simulink model "BD_PAR"  (Simulink 10.1)
settings: Solver=ode1  StartTime=0.0  StopTime=max(cyc_mph(:,1))  FixedStep=1  MaxStep=1  RelTol=1e-3  AbsTol=1e-3
undefined symbols (not defined in the file): ess_on, ex_calc, fc_emis, fc_max_trq, fc_trq_scale, vc_idle_bool, vc_idle_spd
libraries: lib_transmission x4, lib_wheel x2, lib_help x2, lib_accessory x2, lib_controls x2, lib_outputs x1, lib_interactive x1, lib_drive_cycle x1, lib_energy_storage x1, lib_exhaust x1, lib_fuel_converter x1, lib_electric_machine x1
settings Model: Creator=mokeefe  LastModifiedBy=sateeshk  ExtModeTrigMode=oneshot  ExtModeArmWhenConnect=off
settings SolverCC: AutoScaleAbsTol=off
settings DataIOCC: SignalLoggingSaveFormat=ModelDataLogs  SaveOutput=off  SaveTime=off
settings OptimizationCC: BooleanDataType=off  ExpressionDepthLimit=2147483647
settings DebuggingCC: SaveWithParameterizedLinksMsg=none  SignalResolutionControl=TryResolveAllWithWarning  MultiTaskDSMMsg=warning  MultiTaskCondExecSysMsg=none  FcnCallInpInsideContextMsg=warning  UnconnectedLineMsg=none  StateNameClashWarn=warning
settings HardwareCC: TargetUnknown=on
settings RTWCC: TemplateMakefile=grt_vc.tmf

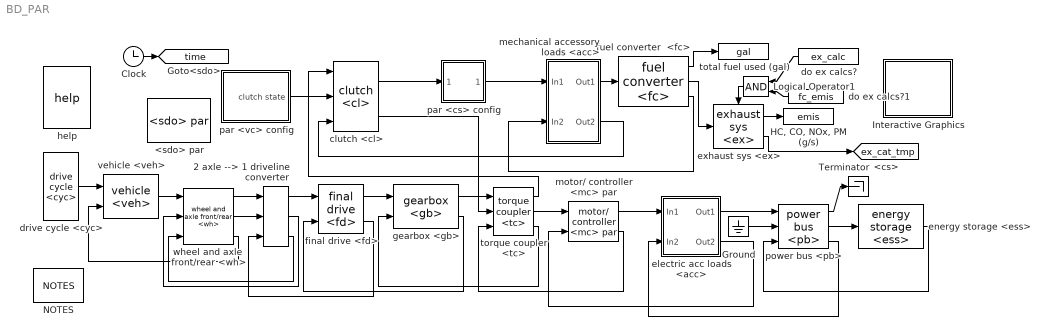
== system BD_PAR ==
  2 axle --> 1 driveline converter : lib_wheel/2 axle --> 1 driveline converter  SystemSampleTime=-1  Latency=0  AutoFrameSizeCalculation=off
  <sdo> par : lib_outputs/<sdo> par  SystemSampleTime=-1  Latency=0  AutoFrameSizeCalculation=off
  Clock : Clock
  Ground : Ground
  "HC, CO, NOx, PM (g/s)" : ToWorkspace  VariableName=emis
  Interactive Graphics : Subsystem  BlockChoice=off
      settings: AttributesFormatString=%<BlockChoice>  TemplateBlock=lib_interactive/Interactive Graphics  MemberBlocks=off,on
  Logical Operator1 : Logic
  NOTES : lib_help/NOTES  SystemSampleTime=-1  Latency=0  AutoFrameSizeCalculation=off
  Terminator : Terminator
  clutch <cl> : lib_transmission/clutch <cl>  slip_spd=vc_launch_spd  maxtrq=max(fc_max_trq)*fc_trq_scale
  do ex calcs? : Constant  Value=ex_calc
  do ex calcs?1 : Constant  Value=fc_emis
  drive cycle <cyc> : lib_drive_cycle/drive cycle <cyc>  SystemSampleTime=-1  Latency=0  AutoFrameSizeCalculation=off
  electric acc loads <acc> : Subsystem
      mask Display: image(imread('bdi_acc_elec.bmp'))
  energy storage <ess> : lib_energy_storage/energy storage <ess>  SystemSampleTime=-1  Latency=0  AutoFrameSizeCalculation=off
      link override ess config: BlockChoice=energy storage <ess>
  exhaust sys <ex> : lib_exhaust/exhaust sys <ex>  SystemSampleTime=-1  Latency=0  AutoFrameSizeCalculation=off
  final drive <fd> : lib_transmission/final drive <fd>  SystemSampleTime=-1  Latency=0  AutoFrameSizeCalculation=off
  fuel converter  <fc> : lib_fuel_converter/fuel converter  <fc>  SystemSampleTime=-1  Latency=0  AutoFrameSizeCalculation=off
      link override fuel use and EO emis Configurable Subsystem: BlockChoice=fuel use and EO emis
  gearbox <gb> : lib_transmission/gearbox <gb>  SystemSampleTime=-1  Latency=0  AutoFrameSizeCalculation=off
  help : lib_help/help  SystemSampleTime=-1  Latency=0  AutoFrameSizeCalculation=off
  mechanical accessory loads <acc> : Subsystem
      mask Display: image(imread('bdi_acc_pic.bmp'))
  motor/ controller <mc> par : lib_electric_machine/motor// controller <mc> par  SystemSampleTime=-1  Latency=0  AutoFrameSizeCalculation=off
  par <cs> config : Subsystem  BlockChoice=electric assist control strategy <cs>
      settings: AttributesFormatString=%<BlockChoice>  TemplateBlock=lib_controls/par <cs> config  MemberBlocks=Adaptive control strategy <cs>,Fuzzy Logic control strategy <cs>,Fuzzy Logic control strategy with Emissions <cs>,electric assist control strategy <cs>,electric assist control strategy bal <cs>
  par <vc> config : Subsystem  BlockChoice=<vc> par
      link override <vc> par Adaptive/config traction control: BlockChoice=traction control
      link override <vc> par/config traction control: BlockChoice=traction control 2 axle
      settings: AttributesFormatString=%<BlockChoice>  TemplateBlock=lib_controls/par <vc> config  MemberBlocks=<vc> par,<vc> par Adaptive,<vc> par balanced
  power bus <pb> : lib_power_bus/power bus <pb>  SystemSampleTime=-1  Latency=0  AutoFrameSizeCalculation=off
  torque coupler <tc> : lib_transmission/torque coupler <tc>  SystemSampleTime=-1  Latency=0  AutoFrameSizeCalculation=off
  total fuel used (gal) : ToWorkspace  VariableName=gal
  vehicle <veh> : lib_vehicle/vehicle <veh>  SystemSampleTime=-1  Latency=0  AutoFrameSizeCalculation=off
      link override record achieved force outputs/rolling resistance force: BlockChoice=force req'd to overcome rolling resistance (N)
      link override rolling resistance force: BlockChoice=force req'd to overcome rolling resistance (N)
      link override vehicle speed: BlockChoice=vehicle speed (m/s)
  wheel and axle  front/rear <wh> : lib_wheel/wheel and axle  front//rear <wh>  SystemSampleTime=-1  Latency=0  AutoFrameSizeCalculation=off
  tag scope: ex_cat_tmp=global, time=global
  wires:
  wheel and axle  front/rear <wh>/3 -> vehicle <veh>/2
  final drive <fd>/2 -> 2 axle --> 1 driveline converter/3
  final drive <fd>/1 -> gearbox <gb>/1
  drive cycle <cyc>/1 -> vehicle <veh>/1
  clutch <cl>/1 -> par <cs> config/1("trq and spd req'd into clutch (N*m, rad/s)")
  fuel converter  <fc>/2 -> exhaust sys <ex>/1
  do ex calcs?/1 -> Logical Operator1/1
  fuel converter  <fc>/1 -> total fuel used (gal)/1
  exhaust sys <ex>/1 -> "HC, CO, NOx, PM (g/s)"/1
  Logical Operator1/1 -> exhaust sys <ex>/Enable
  do ex calcs?1/1 -> Logical Operator1/2
  Clock/1 -> [time]
  gearbox <gb>/2 -> final drive <fd>/2
  torque coupler <tc>/3 -> gearbox <gb>/2
  torque coupler <tc>/1 -> clutch <cl>/1
  clutch <cl>/2 -> torque coupler <tc>/2
  gearbox <gb>/1 -> torque coupler <tc>/1
  par <vc> config/1(clutch state) -> clutch <cl>/2
  motor/ controller <mc> par/2 -> torque coupler <tc>/3
  Ground/1 -> power bus <pb>/2
  power bus <pb>/2 -> energy storage <ess>/1
  power bus <pb>/1 -> Terminator/1
  energy storage <ess>/1 -> power bus <pb>/3
  torque coupler <tc>/2 -> motor/ controller <mc> par/1
  exhaust sys <ex>/2 -> [ex_cat_tmp]
  motor/ controller <mc> par/1 -> electric acc loads <acc>/1(In1)
  electric acc loads <acc>/1(Out1) -> power bus <pb>/1
  power bus <pb>/3 -> electric acc loads <acc>/2(In2)
  electric acc loads <acc>/2(Out2) -> motor/ controller <mc> par/2
  par <cs> config/1("trq and spd req'd from engine (N*m, rad/s)") -> mechanical accessory loads <acc>/1(In1)
  mechanical accessory loads <acc>/1(Out1) -> fuel converter  <fc>/1
  fuel converter  <fc>/3 -> mechanical accessory loads <acc>/2(In2)
  mechanical accessory loads <acc>/2(Out2) -> clutch <cl>/3
  vehicle <veh>/1 -> wheel and axle  front/rear <wh>/1
  wheel and axle  front/rear <wh>/1 -> 2 axle --> 1 driveline converter/1
  wheel and axle  front/rear <wh>/2 -> 2 axle --> 1 driveline converter/2
  2 axle --> 1 driveline converter/2 -> wheel and axle  front/rear <wh>/2
  2 axle --> 1 driveline converter/3 -> wheel and axle  front/rear <wh>/3
  2 axle --> 1 driveline converter/1 -> final drive <fd>/1

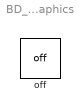
== system BD_PAR/Interactive Graphics ==
  off : lib_interactive/off  Tag=Altia_off  SystemSampleTime=-1  Latency=0  AutoFrameSizeCalculation=off

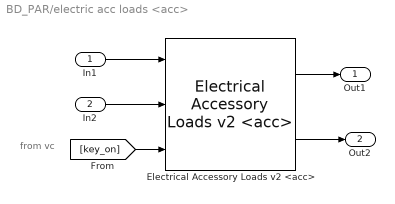
== system BD_PAR/electric acc loads <acc> ==
  note: from vc
  In1 : Inport
  In2 : Inport  Port=2
  Electrical Accessory Loads v2 <acc> : lib_accessory/Electrical Accessory Loads v2 <acc>  load_on=ess_on
      link override backward model/electrical accessories (W): BlockChoice=Electrical Accessories: Time Variable
  Out1 : Outport
  Out2 : Outport  Port=2
  wires:
  In1/1 -> Electrical Accessory Loads v2 <acc>/1
  In2/1 -> Electrical Accessory Loads v2 <acc>/2
  Electrical Accessory Loads v2 <acc>/1 -> Out1/1
  Electrical Accessory Loads v2 <acc>/2 -> Out2/1
  [key_on] -> Electrical Accessory Loads v2 <acc>/3

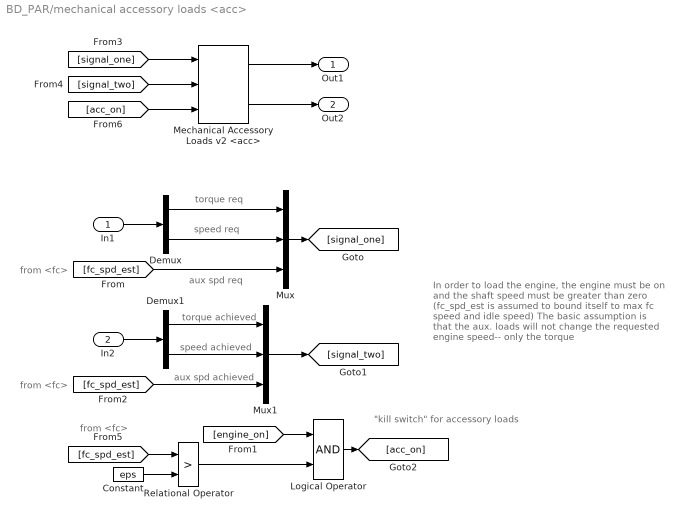
== system BD_PAR/mechanical accessory loads <acc> ==
  note: from <fc>
  note: from <fc>
  note: torque req
  note: speed req
  note: aux spd req
  note: torque achieved
  note: speed achieved
  note: aux spd achieved
  note: from <fc>
  note: In order to load the engine,
      | the engine must be on and
      | the shaft speed must
      | be greater than zero (fc_spd_est is assumed
      | to bound itself to max fc speed and idle speed)
      |
      | The basic assumption is that the aux. loads
      | will not change the requested engine speed--
      | only the torque
  note: "kill switch" for accessory loads
  In1 : Inport
  In2 : Inport  Port=2
  Constant : Constant  Value=eps
  Demux : Demux  Outputs=2
      settings: DisplayOption=none
  Demux1 : Demux  Outputs=2
      settings: DisplayOption=none
  Logical Operator : Logic
  Mechanical Accessory Loads v2 <acc> : lib_accessory/Mechanical Accessory Loads v2 <acc>  load_on=not(ess_on)*1  acc_max_spd=inf  acc_min_spd=vc_idle_spd*vc_idle_bool+eps  ic_mech_trq=0  ic_mech_pwr=0
      link override backward model/mechanical accessories (Nm): BlockChoice=Mechanical Accessories: Const Mech Var Elect
  Mux : Mux  Inputs=3
  Mux1 : Mux  Inputs=3
  Relational Operator : RelationalOperator  Operator=>  RndMeth=Nearest  InputSameDT=on
  Out1 : Outport
  Out2 : Outport  Port=2
  wires:
  [signal_one] -> Mechanical Accessory Loads v2 <acc>/1
  Mechanical Accessory Loads v2 <acc>/1 -> Out1/1
  Mechanical Accessory Loads v2 <acc>/2 -> Out2/1
  [signal_two] -> Mechanical Accessory Loads v2 <acc>/2
  Mux/1 -> [signal_one]
  In1/1 -> Demux/1
  Demux/1 -> Mux/1
  Demux/2 -> Mux/2
  [fc_spd_est] -> Mux/3
  Mux1/1 -> [signal_two]
  In2/1 -> Demux1/1
  Demux1/1 -> Mux1/1
  Demux1/2 -> Mux1/2
  [fc_spd_est] -> Mux1/3
  [engine_on] -> Logical Operator/1
  Logical Operator/1 -> [acc_on]
  [acc_on] -> Mechanical Accessory Loads v2 <acc>/3
  [fc_spd_est] -> Relational Operator/1
  Constant/1 -> Relational Operator/2
  Relational Operator/1 -> Logical Operator/2

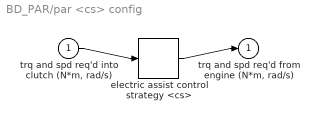
== system BD_PAR/par <cs> config ==
  "trq and spd req'd into clutch (N*m, rad/s)" : Inport
  electric assist control strategy <cs> : lib_controls/electric assist control strategy <cs>  SystemSampleTime=-1  Latency=0  AutoFrameSizeCalculation=off
  "trq and spd req'd from engine (N*m, rad/s)" : Outport
  wires:
  "trq and spd req'd into clutch (N*m, rad/s)"/1 -> electric assist control strategy <cs>/1
  electric assist control strategy <cs>/1 -> "trq and spd req'd from engine (N*m, rad/s)"/1

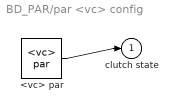
== system BD_PAR/par <vc> config ==
  <vc> par : lib_controls/<vc> par  SystemSampleTime=-1  Latency=0  AutoFrameSizeCalculation=off
  clutch state : Outport
  wires:
  <vc> par/1 -> clutch state/1
